simulink model "ModelN_SMC"  (R2022b)
settings: Solver=ode45  StartTime=0.0  StopTime=50
values from neighbouring files (symbols this model uses):
  Ix = 7.5e-3    (= 0.0075)    [values_1.m]
  Iy = Ix    (= 0.0075)    [values_1.m]
  Iz = 1.3e-2    (= 0.013)    [values_1.m]
  l = 1    [values_1.m]
  lamd1 = -1    [values_1.m]
  lamd2 = 2    [values_1.m]
  lamd3 = 5    [values_1.m]
libraries: simulink x9, slpidlib x3
settings Model: Creator=kumar  LastModifiedBy=Niku

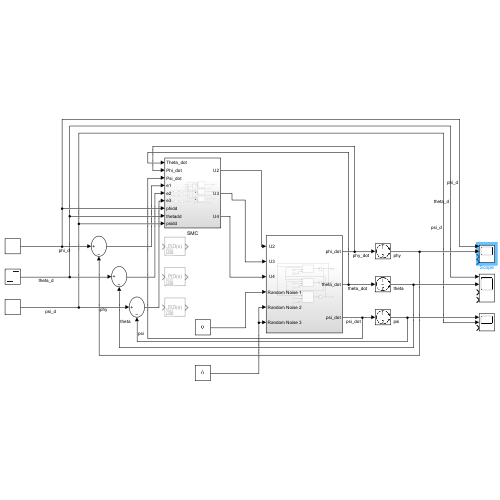
[thumbnail: Simulink's stored preview of the top-level diagram]
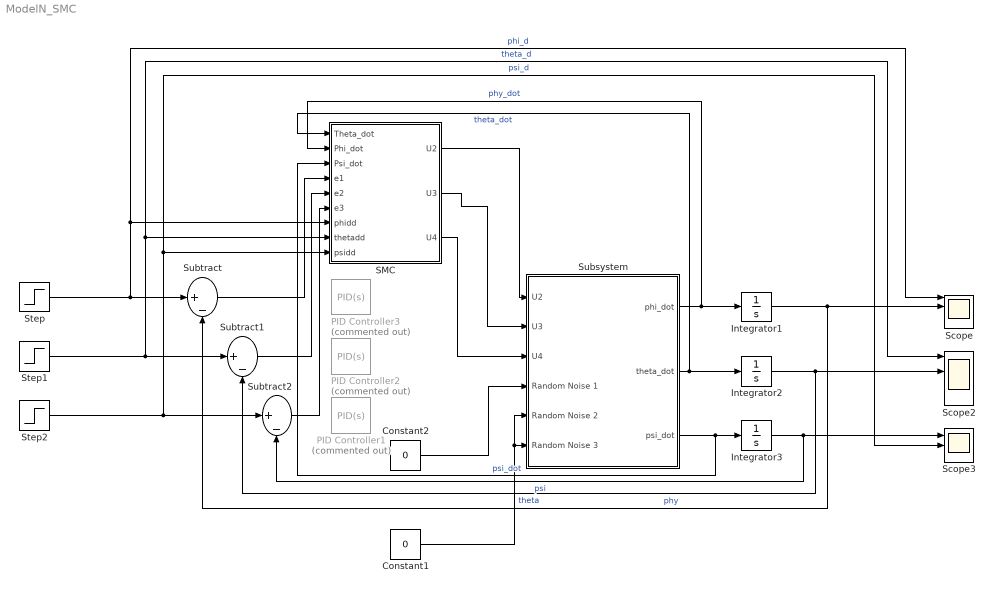
== system ModelN_SMC ==
  Constant1 : Constant  Value=0
  Constant2 : Constant  Value=0
  Integrator1 : Integrator  WrapState=on
  Integrator2 : Integrator  WrapState=on
  Integrator3 : Integrator  WrapState=on
  PID Controller1 : slpidlib/PID Controller  Commented=on  Controller=PID  Form=Parallel  TimeDomain=Continuous-time  UseExternalTs=off  SampleTime=-1  IntegratorMethod=Forward Euler  FilterMethod=Forward Euler  ControllerParametersSource=internal  P=-0.00241383042252482  I=-0.000113002936035472  UseKiTs=off  D=-0.0126609727607765  N=5.45397025421619  UseFilter=on  TunerSelectOption=Transfer Function Based (PID Tuner App)  InitialConditionSource=internal  InitialConditionForIntegrator=0  InitialConditionForFilter=0  DifferentiatorICPrevScaledInput=0  ExternalReset=none  TrackingMode=off  Kt=1  LimitOutput=off  SatLimitsSource=internal  UpperSaturationLimit=inf  LowerSaturationLimit=-inf  LinearizeAsGain=on  AntiWindupMode=none  Kb=1  LimitIntegrator=off  UpperIntegratorSaturationLimit=inf  LowerIntegratorSaturationLimit=-inf  POutMin=[]  POutMax=[]  IOutMin=[]  IOutMax=[]  DOutMin=[]  DOutMax=[]  NOutMin=[]  NOutMax=[]  SumOutMin=[]  SumOutMax=[]  SaturationOutMin=[]  SaturationOutMax=[]  PParamMin=[]  PParamMax=[]  IParamMin=[]  IParamMax=[]  DParamMin=[]  DParamMax=[]  NParamMin=[]  NParamMax=[]  KbParamMin=[]  KbParamMax=[]  KtParamMin=[]  KtParamMax=[]  KbOutMin=[]  KbOutMax=[]  KtOutMin=[]  KtOutMax=[]  IntegratorOutMin=[]  IntegratorOutMax=[]  FilterOutMin=[]  FilterOutMax=[]  SumI1OutMin=[]  SumI1OutMax=[]  SumI2OutMin=[]  SumI2OutMax=[]  SumI3OutMin=[]  SumI3OutMax=[]  SumI4OutMin=[]  SumI4OutMax=[]  SumDOutMin=[]  SumDOutMax=[]  DifferentiatorOutMin=[]  DifferentiatorOutMax=[]  FilterDiffOutCoefMin=[]  FilterDiffOutCoefMax=[]  ReciprocalOutMin=[]  ReciprocalOutMax=[]  SumDenOutMin=[]  SumDenOutMax=[]  SumNumOutMin=[]  SumNumOutMax=[]  DivideOutMin=[]  DivideOutMax=[]  UdiffTsProdOutMin=[]  UdiffTsProdOutMax=[]  NTsProdOutMin=[]  NTsProdOutMax=[]  UintegralTsProdOutMin=[]  UintegralTsProdOutMax=[]  UngainTsProdOutMin=[]  UngainTsProdOutMax=[]  ClampingZeroOutDataTypeStr=Inherit: Inherit via back propagation  ClampingZeroOutMin=[]  ClampingZeroOutMax=[]  FilterDenConstantOutDataTypeStr=Inherit: Inherit via back propagation  FilterDenConstantOutMin=[]  FilterDenConstantOutMax=[]  PCopyOutDataTypeStr=Inherit: Inherit via back propagation  PCopyOutMin=[]  PCopyOutMax=[]  NCopyOutDataTypeStr=Inherit: Inherit via back propagation  NCopyOutMin=[]  NCopyOutMax=[]  IntegratorContinuousStateAttributes=''  IntegratorStateMustResolveToSignalObject=off  IntegratorRTWStateStorageClass=Auto  FilterContinuousStateAttributes=''  FilterStateMustResolveToSignalObject=off  FilterRTWStateStorageClass=Auto  ParallelPVariant=InternalParameters  IdealPVariant=Disabled  IVariant=InternalParameters  DVariant=InternalParameters  IntegratorVariant=Continuous  SatVariant=Disabled  AWVariant=Passthrough  PCopyVariant=Disabled  TRVariant=Disabled  FdbkBlocksVariant=Forward  IdealPFdbkVariant=Disabled  SatFdbkVariant=Disabled  DerivativeFilterVariant=ContFilter  NVariant=InternalParameters  NCopyVariant=Disabled  FilterICVariant=InternalICsFilter  IntegratorICVariant=InternalICs  ExternalResetVariant=Disabled  TRSumVariant=Passthrough  SumFdbkVariant=Disabled  SumVariant=Sum_PID  TsampFilterVariant=InternalTs  TsampNgainVariant=Passthrough  TsampIntegralVariant=Passthrough  ExternalSaturationOutDataTypeStr=Inherit: Same as second input
  PID Controller2 : slpidlib/PID Controller  Commented=on  Controller=PID  Form=Parallel  TimeDomain=Continuous-time  UseExternalTs=off  SampleTime=-1  IntegratorMethod=Forward Euler  FilterMethod=Forward Euler  ControllerParametersSource=internal  P=-0.00605475858492847  I=-0.000283452180690982  UseKiTs=off  D=-0.031758292878202  N=5.45397025421619  UseFilter=on  TunerSelectOption=Transfer Function Based (PID Tuner App)  InitialConditionSource=internal  InitialConditionForIntegrator=0  InitialConditionForFilter=0  DifferentiatorICPrevScaledInput=0  ExternalReset=none  TrackingMode=off  Kt=1  LimitOutput=off  SatLimitsSource=internal  UpperSaturationLimit=inf  LowerSaturationLimit=-inf  LinearizeAsGain=on  AntiWindupMode=none  Kb=1  LimitIntegrator=off  UpperIntegratorSaturationLimit=inf  LowerIntegratorSaturationLimit=-inf  POutMin=[]  POutMax=[]  IOutMin=[]  IOutMax=[]  DOutMin=[]  DOutMax=[]  NOutMin=[]  NOutMax=[]  SumOutMin=[]  SumOutMax=[]  SaturationOutMin=[]  SaturationOutMax=[]  PParamMin=[]  PParamMax=[]  IParamMin=[]  IParamMax=[]  DParamMin=[]  DParamMax=[]  NParamMin=[]  NParamMax=[]  KbParamMin=[]  KbParamMax=[]  KtParamMin=[]  KtParamMax=[]  KbOutMin=[]  KbOutMax=[]  KtOutMin=[]  KtOutMax=[]  IntegratorOutMin=[]  IntegratorOutMax=[]  FilterOutMin=[]  FilterOutMax=[]  SumI1OutMin=[]  SumI1OutMax=[]  SumI2OutMin=[]  SumI2OutMax=[]  SumI3OutMin=[]  SumI3OutMax=[]  SumI4OutMin=[]  SumI4OutMax=[]  SumDOutMin=[]  SumDOutMax=[]  DifferentiatorOutMin=[]  DifferentiatorOutMax=[]  FilterDiffOutCoefMin=[]  FilterDiffOutCoefMax=[]  ReciprocalOutMin=[]  ReciprocalOutMax=[]  SumDenOutMin=[]  SumDenOutMax=[]  SumNumOutMin=[]  SumNumOutMax=[]  DivideOutMin=[]  DivideOutMax=[]  UdiffTsProdOutMin=[]  UdiffTsProdOutMax=[]  NTsProdOutMin=[]  NTsProdOutMax=[]  UintegralTsProdOutMin=[]  UintegralTsProdOutMax=[]  UngainTsProdOutMin=[]  UngainTsProdOutMax=[]  ClampingZeroOutDataTypeStr=Inherit: Inherit via back propagation  ClampingZeroOutMin=[]  ClampingZeroOutMax=[]  FilterDenConstantOutDataTypeStr=Inherit: Inherit via back propagation  FilterDenConstantOutMin=[]  FilterDenConstantOutMax=[]  PCopyOutDataTypeStr=Inherit: Inherit via back propagation  PCopyOutMin=[]  PCopyOutMax=[]  NCopyOutDataTypeStr=Inherit: Inherit via back propagation  NCopyOutMin=[]  NCopyOutMax=[]  IntegratorContinuousStateAttributes=''  IntegratorStateMustResolveToSignalObject=off  IntegratorRTWStateStorageClass=Auto  FilterContinuousStateAttributes=''  FilterStateMustResolveToSignalObject=off  FilterRTWStateStorageClass=Auto  ParallelPVariant=InternalParameters  IdealPVariant=Disabled  IVariant=InternalParameters  DVariant=InternalParameters  IntegratorVariant=Continuous  SatVariant=Disabled  AWVariant=Passthrough  PCopyVariant=Disabled  TRVariant=Disabled  FdbkBlocksVariant=Forward  IdealPFdbkVariant=Disabled  SatFdbkVariant=Disabled  DerivativeFilterVariant=ContFilter  NVariant=InternalParameters  NCopyVariant=Disabled  FilterICVariant=InternalICsFilter  IntegratorICVariant=InternalICs  ExternalResetVariant=Disabled  TRSumVariant=Passthrough  SumFdbkVariant=Disabled  SumVariant=Sum_PID  TsampFilterVariant=InternalTs  TsampNgainVariant=Passthrough  TsampIntegralVariant=Passthrough  ExternalSaturationOutDataTypeStr=Inherit: Same as second input
  PID Controller3 : slpidlib/PID Controller  Commented=on  Controller=PID  Form=Parallel  TimeDomain=Continuous-time  UseExternalTs=off  SampleTime=-1  IntegratorMethod=Forward Euler  FilterMethod=Forward Euler  ControllerParametersSource=internal  P=0.00605475858492847  I=0.000283452180690982  UseKiTs=off  D=0.031758292878202  N=5.45397025421619  UseFilter=on  TunerSelectOption=Transfer Function Based (PID Tuner App)  InitialConditionSource=internal  InitialConditionForIntegrator=0  InitialConditionForFilter=0  DifferentiatorICPrevScaledInput=0  ExternalReset=none  TrackingMode=off  Kt=1  LimitOutput=off  SatLimitsSource=internal  UpperSaturationLimit=inf  LowerSaturationLimit=-inf  LinearizeAsGain=on  AntiWindupMode=none  Kb=1  LimitIntegrator=off  UpperIntegratorSaturationLimit=inf  LowerIntegratorSaturationLimit=-inf  POutMin=[]  POutMax=[]  IOutMin=[]  IOutMax=[]  DOutMin=[]  DOutMax=[]  NOutMin=[]  NOutMax=[]  SumOutMin=[]  SumOutMax=[]  SaturationOutMin=[]  SaturationOutMax=[]  PParamMin=[]  PParamMax=[]  IParamMin=[]  IParamMax=[]  DParamMin=[]  DParamMax=[]  NParamMin=[]  NParamMax=[]  KbParamMin=[]  KbParamMax=[]  KtParamMin=[]  KtParamMax=[]  KbOutMin=[]  KbOutMax=[]  KtOutMin=[]  KtOutMax=[]  IntegratorOutMin=[]  IntegratorOutMax=[]  FilterOutMin=[]  FilterOutMax=[]  SumI1OutMin=[]  SumI1OutMax=[]  SumI2OutMin=[]  SumI2OutMax=[]  SumI3OutMin=[]  SumI3OutMax=[]  SumI4OutMin=[]  SumI4OutMax=[]  SumDOutMin=[]  SumDOutMax=[]  DifferentiatorOutMin=[]  DifferentiatorOutMax=[]  FilterDiffOutCoefMin=[]  FilterDiffOutCoefMax=[]  ReciprocalOutMin=[]  ReciprocalOutMax=[]  SumDenOutMin=[]  SumDenOutMax=[]  SumNumOutMin=[]  SumNumOutMax=[]  DivideOutMin=[]  DivideOutMax=[]  UdiffTsProdOutMin=[]  UdiffTsProdOutMax=[]  NTsProdOutMin=[]  NTsProdOutMax=[]  UintegralTsProdOutMin=[]  UintegralTsProdOutMax=[]  UngainTsProdOutMin=[]  UngainTsProdOutMax=[]  ClampingZeroOutDataTypeStr=Inherit: Inherit via back propagation  ClampingZeroOutMin=[]  ClampingZeroOutMax=[]  FilterDenConstantOutDataTypeStr=Inherit: Inherit via back propagation  FilterDenConstantOutMin=[]  FilterDenConstantOutMax=[]  PCopyOutDataTypeStr=Inherit: Inherit via back propagation  PCopyOutMin=[]  PCopyOutMax=[]  NCopyOutDataTypeStr=Inherit: Inherit via back propagation  NCopyOutMin=[]  NCopyOutMax=[]  IntegratorContinuousStateAttributes=''  IntegratorStateMustResolveToSignalObject=off  IntegratorRTWStateStorageClass=Auto  FilterContinuousStateAttributes=''  FilterStateMustResolveToSignalObject=off  FilterRTWStateStorageClass=Auto  ParallelPVariant=InternalParameters  IdealPVariant=Disabled  IVariant=InternalParameters  DVariant=InternalParameters  IntegratorVariant=Continuous  SatVariant=Disabled  AWVariant=Passthrough  PCopyVariant=Disabled  TRVariant=Disabled  FdbkBlocksVariant=Forward  IdealPFdbkVariant=Disabled  SatFdbkVariant=Disabled  DerivativeFilterVariant=ContFilter  NVariant=InternalParameters  NCopyVariant=Disabled  FilterICVariant=InternalICsFilter  IntegratorICVariant=InternalICs  ExternalResetVariant=Disabled  TRSumVariant=Passthrough  SumFdbkVariant=Disabled  SumVariant=Sum_PID  TsampFilterVariant=InternalTs  TsampNgainVariant=Passthrough  TsampIntegralVariant=Passthrough  ExternalSaturationOutDataTypeStr=Inherit: Same as second input
  SMC : Subsystem
  Scope : Scope  NumInputPorts=4
  Scope2 : Scope  NumInputPorts=4
  Scope3 : Scope  NumInputPorts=3
  Step : Step  SampleTime=0
  Step1 : Step  After=2  SampleTime=0
  Step2 : Step  After=3  SampleTime=0
  Subsystem : Subsystem
  Subtract : Sum  Inputs=|+-
  Subtract1 : Sum  Inputs=|+-
  Subtract2 : Sum  Inputs=|+-
  wires:
  Subsystem/1(phi_dot) -> SMC/2(Phi_dot), Integrator1/1  "phy_dot"
  Subsystem/2(theta_dot) -> Integrator2/1, SMC/1(Theta_dot)  "theta_dot"
  Subsystem/3(psi_dot) -> Integrator3/1, SMC/3(Psi_dot)  "psi_dot"
  Integrator1/1 -> Scope/2, Subtract/2  "phy"
  Integrator2/1 -> Scope2/2, Subtract1/2  "theta"
  Integrator3/1 -> Scope3/1, Subtract2/2  "psi"
  Constant1/1 -> Subsystem/5(Random Noise 2), Subsystem/6(Random Noise 3)
  Constant2/1 -> Subsystem/4(Random Noise 1)
  Step/1 -> Subtract/1, SMC/7(phidd), Scope/1  "phi_d"
  Step1/1 -> Subtract1/1, SMC/8(thetadd), Scope2/1  "theta_d"
  Subtract2/1 -> SMC/6(e3)
  Step2/1 -> Subtract2/1, SMC/9(psidd), Scope3/2  "psi_d"
  Subtract1/1 -> SMC/5(e2)
  Subtract/1 -> SMC/4(e1)
  SMC/3(U4) -> Subsystem/3(" U4")
  SMC/2(U3) -> Subsystem/2(" U3")
  SMC/1(U2) -> Subsystem/1(" U2")

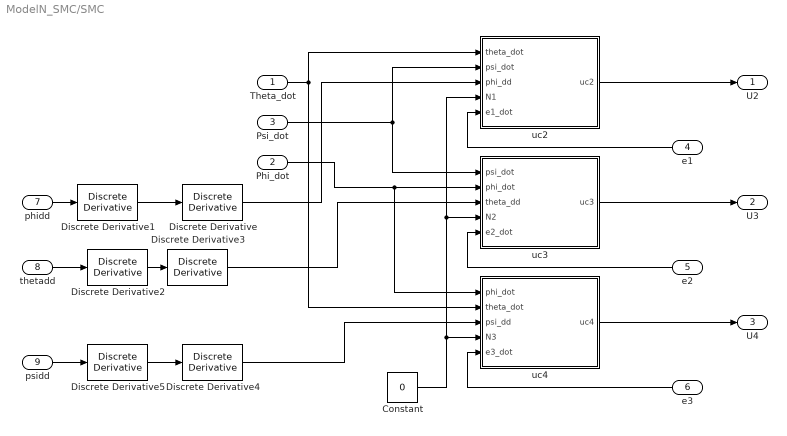
== system ModelN_SMC/SMC ==
  Theta_dot : Inport
  Phi_dot : Inport  Port=2
  Psi_dot : Inport  Port=3
  e1 : Inport  Port=4
  e2 : Inport  Port=5
  e3 : Inport  Port=6
  phidd : Inport  Port=7
  thetadd : Inport  Port=8
  psidd : Inport  Port=9
  Constant : Constant  Value=0
  Discrete Derivative : simulink/Discrete/Discrete Derivative  gainval=1  ICPrevScaledInput=0.0  OutMin=[]  OutMax=[]  OutDataType=fixdt(1, 16)  OutScaling=2^-10  DoSatur=off
  Discrete Derivative1 : simulink/Discrete/Discrete Derivative  gainval=1  ICPrevScaledInput=0.0  OutMin=[]  OutMax=[]  OutDataType=fixdt(1, 16)  OutScaling=2^-10  DoSatur=off
  Discrete Derivative{2..5} (4 alike) : simulink/Discrete/Discrete Derivative  gainval=1.0  ICPrevScaledInput=0.0  OutMin=[]  OutMax=[]  OutDataType=fixdt(1, 16)  OutScaling=2^-10  DoSatur=off
  uc2 : Subsystem
  uc3 : Subsystem
  uc4 : Subsystem
  U2 : Outport
  U3 : Outport  Port=2
  U4 : Outport  Port=3
  wires:
  uc2/1(uc2) -> U2/1
  uc4/1(uc4) -> U4/1
  uc3/1(uc3) -> U3/1
  Theta_dot/1 -> uc2/1(theta_dot), uc4/2(theta_dot)
  Phi_dot/1 -> uc3/2(phi_dot), uc4/1(phi_dot)
  Psi_dot/1 -> uc3/1(psi_dot), uc2/2(psi_dot)
  Constant/1 -> uc4/4(N3), uc2/4(N1), uc3/4(N2)
  e1/1 -> uc2/5(e1_dot)
  e2/1 -> uc3/5(e2_dot)
  e3/1 -> uc4/5(e3_dot)
  Discrete Derivative3/1 -> uc3/3(theta_dd)
  phidd/1 -> Discrete Derivative1/1
  Discrete Derivative1/1 -> Discrete Derivative/1
  psidd/1 -> Discrete Derivative5/1
  thetadd/1 -> Discrete Derivative2/1
  Discrete Derivative2/1 -> Discrete Derivative3/1
  Discrete Derivative5/1 -> Discrete Derivative4/1
  Discrete Derivative/1 -> uc2/3(phi_dd)
  Discrete Derivative4/1 -> uc4/3(psi_dd)

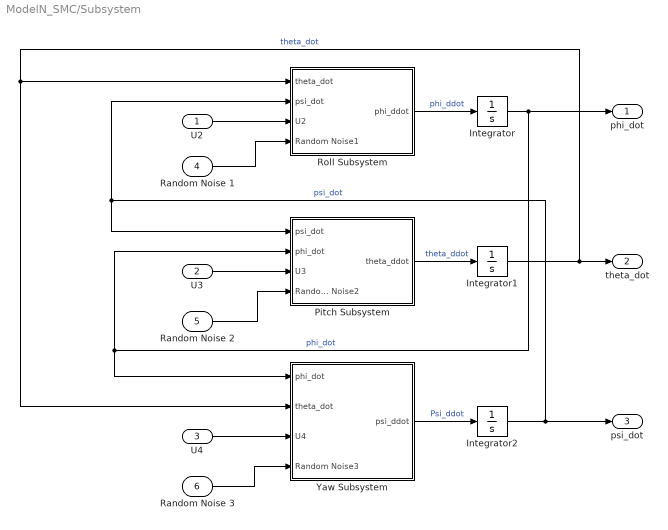
== system ModelN_SMC/Subsystem ==
  " U2" : Inport
  " U3" : Inport  Port=2
  " U4" : Inport  Port=3
  Random Noise 1 : Inport  Port=4
  Random Noise 2 : Inport  Port=5
  Random Noise 3 : Inport  Port=6
  Integrator : Integrator
  Integrator1 : Integrator
  Integrator2 : Integrator
  Pitch Subsystem : Subsystem
  Roll Subsystem : Subsystem
  Yaw Subsystem : Subsystem
  phi_dot : Outport
  theta_dot : Outport  Port=2
  psi_dot : Outport  Port=3
  wires:
  " U2"/1 -> Roll Subsystem/3(" U2")
  Random Noise 1/1 -> Roll Subsystem/4(Random Noise1)
  Yaw Subsystem/1(psi_ddot) -> Integrator2/1  "Psi_ddot"
  " U3"/1 -> Pitch Subsystem/3(" U3")
  Random Noise 2/1 -> Pitch Subsystem/4(Random Noise2)
  " U4"/1 -> Yaw Subsystem/3(" U4")
  Random Noise 3/1 -> Yaw Subsystem/4(Random Noise3)
  Roll Subsystem/1(phi_ddot) -> Integrator/1  "phi_ddot"
  Pitch Subsystem/1(theta_ddot) -> Integrator1/1  "theta_ddot"
  Integrator/1 -> Yaw Subsystem/1(phi_dot), Pitch Subsystem/2(phi_dot), phi_dot/1  "phi_dot"
  Integrator1/1 -> theta_dot/1, Yaw Subsystem/2(theta_dot), Roll Subsystem/1(theta_dot)  "theta_dot"
  Integrator2/1 -> Pitch Subsystem/1(psi_dot), Roll Subsystem/2(psi_dot), psi_dot/1  "psi_dot"

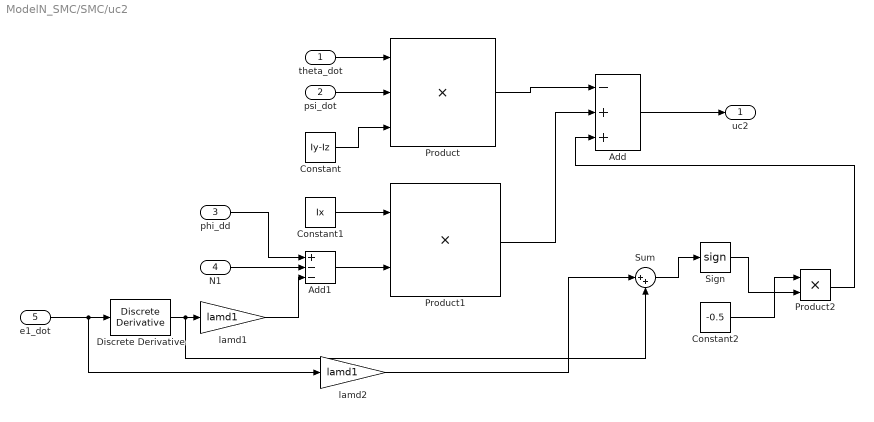
== system ModelN_SMC/SMC/uc2 ==
  theta_dot : Inport
  psi_dot : Inport  Port=2
  phi_dd : Inport  Port=3
  N1 : Inport  Port=4
  e1_dot : Inport  Port=5
  Add : Sum  Inputs=-++
  Add1 : Sum  Inputs=+--
  Constant : Constant  Value=Iy-Iz
  Constant1 : Constant  Value=Ix
  Constant2 : Constant  Value=-0.5
  Discrete Derivative : simulink/Discrete/Discrete Derivative  gainval=1.0  ICPrevScaledInput=0.0  OutMin=[]  OutMax=[]  OutDataType=fixdt(1, 16)  OutScaling=2^-10  DoSatur=off
  Product : Product  Inputs=3
  Product1 : Product
  Product2 : Product
  Sign : Signum
  Sum : Sum  Inputs=|++
  lamd1 : Gain  Gain=lamd1
  lamd2 : Gain  Gain=lamd1
  uc2 : Outport
  wires:
  Constant/1 -> Product/3
  Constant1/1 -> Product1/1
  theta_dot/1 -> Product/1
  psi_dot/1 -> Product/2
  Product/1 -> Add/1
  Add1/1 -> Product1/2
  Product1/1 -> Add/2
  Add/1 -> uc2/1
  phi_dd/1 -> Add1/1
  N1/1 -> Add1/2
  e1_dot/1 -> lamd2/1, Discrete Derivative/1
  lamd1/1 -> Add1/3
  Discrete Derivative/1 -> Sum/2, lamd1/1
  Sum/1 -> Sign/1
  Constant2/1 -> Product2/1
  Sign/1 -> Product2/2
  Product2/1 -> Add/3
  lamd2/1 -> Sum/1

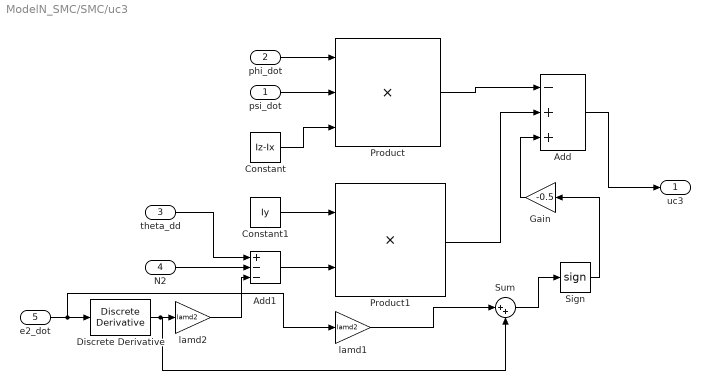
== system ModelN_SMC/SMC/uc3 ==
  psi_dot : Inport
  phi_dot : Inport  Port=2
  theta_dd : Inport  Port=3
  N2 : Inport  Port=4
  e2_dot : Inport  Port=5
  Add : Sum  Inputs=-++
  Add1 : Sum  Inputs=+--
  Constant : Constant  Value=Iz-Ix
  Constant1 : Constant  Value=Iy
  Discrete Derivative : simulink/Discrete/Discrete Derivative  gainval=1.0  ICPrevScaledInput=0.0  OutMin=[]  OutMax=[]  OutDataType=fixdt(1, 16)  OutScaling=2^-10  DoSatur=off
  Gain : Gain  Gain=-0.5
  Product : Product  Inputs=3
  Product1 : Product
  Sign : Signum
  Sum : Sum  Inputs=|++
  lamd1 : Gain  Gain=lamd2
  lamd2 : Gain  Gain=lamd2
  uc3 : Outport
  wires:
  lamd2/1 -> Add1/3
  e2_dot/1 -> lamd1/1, Discrete Derivative/1
  N2/1 -> Add1/2
  theta_dd/1 -> Add1/1
  Add/1 -> uc3/1
  Product1/1 -> Add/2
  Add1/1 -> Product1/2
  Product/1 -> Add/1
  psi_dot/1 -> Product/2
  phi_dot/1 -> Product/1
  Constant1/1 -> Product1/1
  Constant/1 -> Product/3
  Discrete Derivative/1 -> Sum/2, lamd2/1
  Sum/1 -> Sign/1
  Sign/1 -> Gain/1
  Gain/1 -> Add/3
  lamd1/1 -> Sum/1

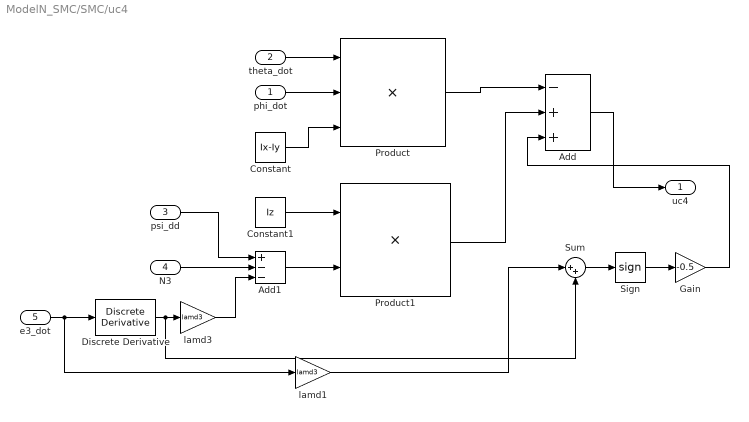
== system ModelN_SMC/SMC/uc4 ==
  phi_dot : Inport
  theta_dot : Inport  Port=2
  psi_dd : Inport  Port=3
  N3 : Inport  Port=4
  e3_dot : Inport  Port=5
  Add : Sum  Inputs=-++
  Add1 : Sum  Inputs=+--
  Constant : Constant  Value=Ix-Iy
  Constant1 : Constant  Value=Iz
  Discrete Derivative : simulink/Discrete/Discrete Derivative  gainval=1.0  ICPrevScaledInput=0.0  OutMin=[]  OutMax=[]  OutDataType=fixdt(1, 16)  OutScaling=2^-10  DoSatur=off
  Gain : Gain  Gain=-0.5
  Product : Product  Inputs=3
  Product1 : Product
  Sign : Signum
  Sum : Sum  Inputs=|++
  lamd1 : Gain  Gain=lamd3
  lamd3 : Gain  Gain=lamd3
  uc4 : Outport
  wires:
  Constant/1 -> Product/3
  Constant1/1 -> Product1/1
  theta_dot/1 -> Product/1
  phi_dot/1 -> Product/2
  Product/1 -> Add/1
  Add1/1 -> Product1/2
  Product1/1 -> Add/2
  Add/1 -> uc4/1
  psi_dd/1 -> Add1/1
  N3/1 -> Add1/2
  e3_dot/1 -> lamd1/1, Discrete Derivative/1
  lamd3/1 -> Add1/3
  Discrete Derivative/1 -> Sum/2, lamd3/1
  Sum/1 -> Sign/1
  Sign/1 -> Gain/1
  Gain/1 -> Add/3
  lamd1/1 -> Sum/1

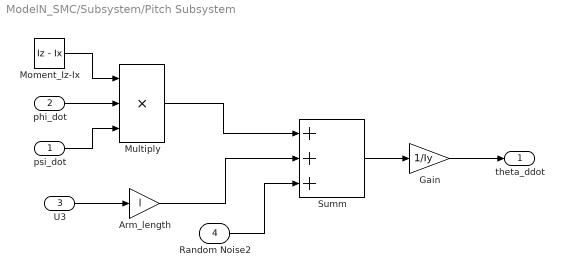
== system ModelN_SMC/Subsystem/Pitch Subsystem ==
  psi_dot : Inport
  phi_dot : Inport  Port=2
  " U3" : Inport  Port=3
  Random Noise2 : Inport  Port=4
  Arm_length : Gain  Gain=l
  Gain : Gain  Gain=1/Iy
  Moment_Iz-Ix : Constant  Value=Iz - Ix
  Multiply : Product  Inputs=3
  Summ : Sum  Inputs=+++
  theta_ddot : Outport
  wires:
  Random Noise2/1 -> Summ/3
  Multiply/1 -> Summ/1
  phi_dot/1 -> Multiply/2
  Arm_length/1 -> Summ/2
  Summ/1 -> Gain/1
  Gain/1 -> theta_ddot/1
  psi_dot/1 -> Multiply/3
  " U3"/1 -> Arm_length/1
  Moment_Iz-Ix/1 -> Multiply/1

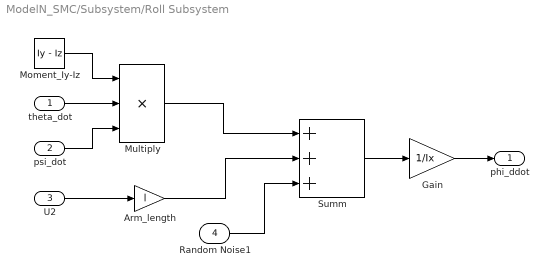
== system ModelN_SMC/Subsystem/Roll Subsystem ==
  theta_dot : Inport
  psi_dot : Inport  Port=2
  " U2" : Inport  Port=3
  Random Noise1 : Inport  Port=4
  Arm_length : Gain  Gain=l
  Gain : Gain  Gain=1/Ix
  Moment_Iy-Iz : Constant  Value=Iy - Iz
  Multiply : Product  Inputs=3
  Summ : Sum  Inputs=+++
  phi_ddot : Outport
  wires:
  Arm_length/1 -> Summ/2
  Gain/1 -> phi_ddot/1
  theta_dot/1 -> Multiply/2
  Multiply/1 -> Summ/1
  Summ/1 -> Gain/1
  " U2"/1 -> Arm_length/1
  psi_dot/1 -> Multiply/3
  Moment_Iy-Iz/1 -> Multiply/1
  Random Noise1/1 -> Summ/3

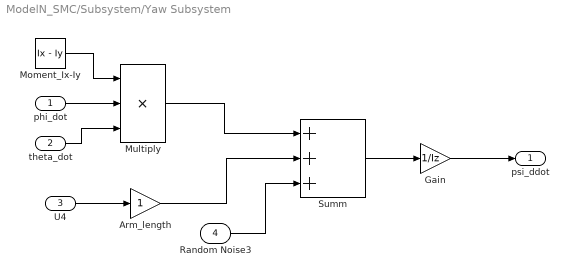
== system ModelN_SMC/Subsystem/Yaw Subsystem ==
  phi_dot : Inport
  theta_dot : Inport  Port=2
  " U4" : Inport  Port=3
  Random Noise3 : Inport  Port=4
  Arm_length : Gain
  Gain : Gain  Gain=1/Iz
  Moment_Ix-Iy : Constant  Value=Ix - Iy
  Multiply : Product  Inputs=3
  Summ : Sum  Inputs=+++
  psi_ddot : Outport
  wires:
  " U4"/1 -> Arm_length/1
  phi_dot/1 -> Multiply/2
  Summ/1 -> Gain/1
  Multiply/1 -> Summ/1
  Gain/1 -> psi_ddot/1
  Arm_length/1 -> Summ/2
  Random Noise3/1 -> Summ/3
  theta_dot/1 -> Multiply/3
  Moment_Ix-Iy/1 -> Multiply/1
